simulink model "Simulinkmodel"  (R2020a)
settings: Solver=VariableStepAuto  StartTime=0.0  StopTime=10.0  RelTol=1e-3
model workspace: external: MAT-File D:\FinalSimulink\fulleasy_DataFile1.mat (data not in the file)
undefined symbols (not defined in the file or in its folder): curveData, height_plane, plane_x, plane_y, smiData, X, Y, Z
libraries: sm_lib x51, Contact_Forces_Lib x48, nesl_utility x36, walkingRobotUtils x8, simulink x1
(part 2 of 2)

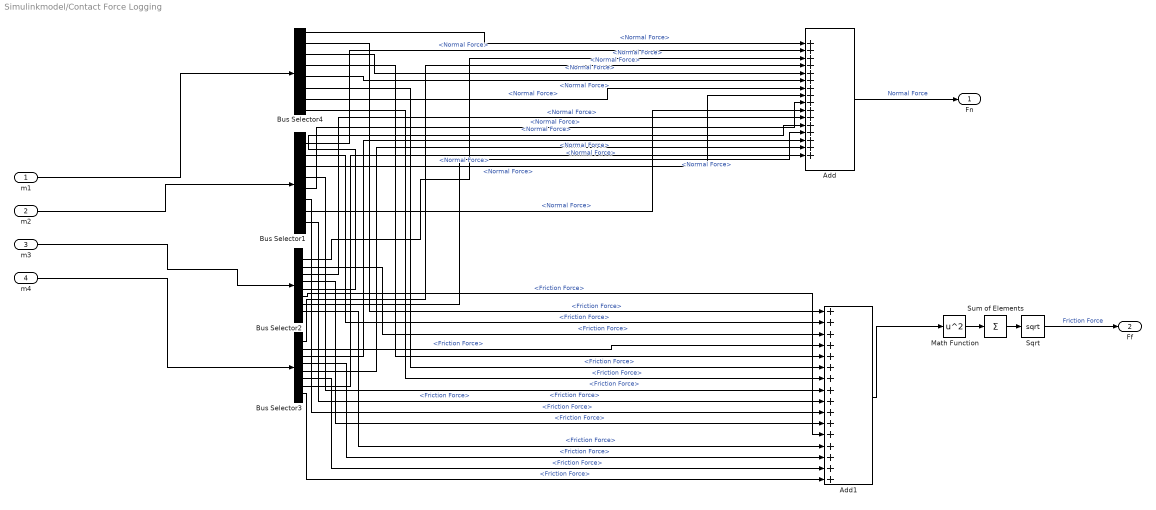
== system Simulinkmodel/Contact Force Logging ==
  m1 : Inport
  m2 : Inport  Port=2
  m3 : Inport  Port=3
  m4 : Inport  Port=4
  Add : Sum  Inputs=16
  Add1 : Sum  Inputs=16
  Bus Selector{1..4} (4 alike) : BusSelector  OutputSignals=fz1.Normal Force,fz1.Friction Force,fz2.Normal Force,fz2.Friction Force,fz3.Normal Force,fz3.Friction Force,fz4.Normal Force,fz4.Friction Force
  Math Function : Math  Operator=square  SignedPower=on  SaturateOnIntegerOverflow=on
  Sqrt : Sqrt  SaturateOnIntegerOverflow=on
  Sum of Elements : Sum  Inputs=+
  Fn : Outport  VectorParamsAs1DForOutWhenUnconnected=off
  Ff : Outport  Port=2  VectorParamsAs1DForOutWhenUnconnected=off
  wires:
  Sqrt/1 -> Ff/1  "Friction Force"
  Sum of Elements/1 -> Sqrt/1
  Math Function/1 -> Sum of Elements/1
  Add1/1 -> Math Function/1
  Add/1 -> Fn/1  "Normal Force"
  Bus Selector3/2 -> Add1/4  "<Friction Force>"
  Bus Selector2/2 -> Add1/3  "<Friction Force>"
  Bus Selector1/2 -> Add1/2  "<Friction Force>"
  Bus Selector4/2 -> Add1/1  "<Friction Force>"
  Bus Selector3/1 -> Add/4  "<Normal Force>"
  Bus Selector2/1 -> Add/3  "<Normal Force>"
  Bus Selector1/1 -> Add/2  "<Normal Force>"
  Bus Selector4/1 -> Add/1  "<Normal Force>"
  m4/1 -> Bus Selector3/1
  m3/1 -> Bus Selector2/1
  m2/1 -> Bus Selector1/1
  m1/1 -> Bus Selector4/1
  Bus Selector4/3 -> Add/5  "<Normal Force>"
  Bus Selector4/4 -> Add1/5  "<Friction Force>"
  Bus Selector4/5 -> Add/6  "<Normal Force>"
  Bus Selector4/6 -> Add1/6  "<Friction Force>"
  Bus Selector4/7 -> Add/7  "<Normal Force>"
  Bus Selector4/8 -> Add1/7  "<Friction Force>"
  Bus Selector1/3 -> Add/8  "<Normal Force>"
  Bus Selector1/4 -> Add1/8  "<Friction Force>"
  Bus Selector1/5 -> Add/9  "<Normal Force>"
  Bus Selector1/6 -> Add1/10  "<Friction Force>"
  Bus Selector1/7 -> Add/10  "<Normal Force>"
  Bus Selector1/8 -> Add1/9  "<Friction Force>"
  Bus Selector2/3 -> Add/11  "<Normal Force>"
  Bus Selector2/4 -> Add1/11  "<Friction Force>"
  Bus Selector2/5 -> Add/12  "<Normal Force>"
  Bus Selector2/6 -> Add1/12  "<Friction Force>"
  Bus Selector2/7 -> Add/13  "<Normal Force>"
  Bus Selector2/8 -> Add1/13  "<Friction Force>"
  Bus Selector3/3 -> Add/14  "<Normal Force>"
  Bus Selector3/4 -> Add1/14  "<Friction Force>"
  Bus Selector3/5 -> Add/15  "<Normal Force>"
  Bus Selector3/6 -> Add1/15  "<Friction Force>"
  Bus Selector3/7 -> Add/16  "<Normal Force>"
  Bus Selector3/8 -> Add1/16  "<Friction Force>"

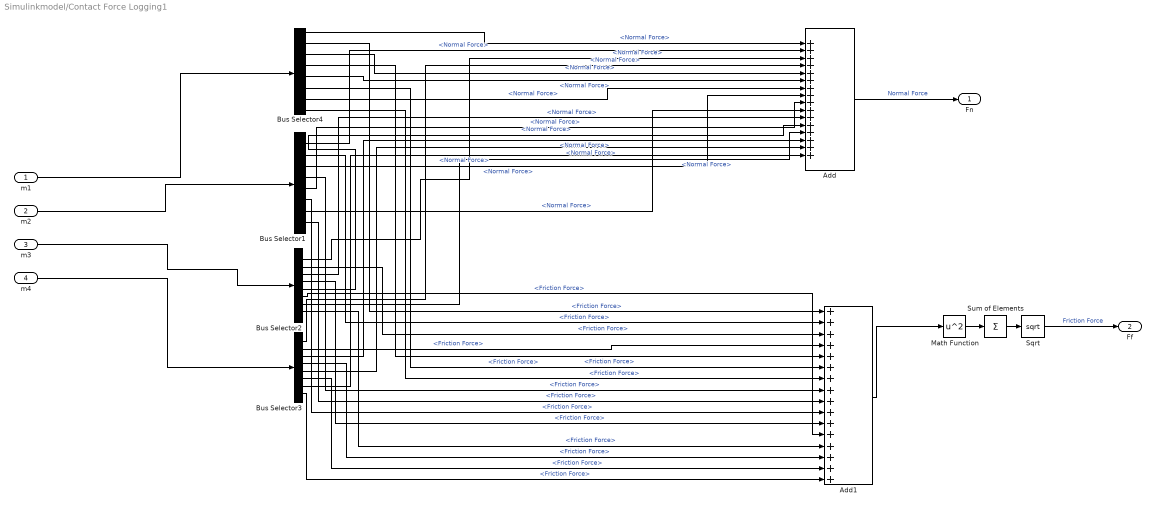
== system Simulinkmodel/Contact Force Logging1 ==
  m1 : Inport
  m2 : Inport  Port=2
  m3 : Inport  Port=3
  m4 : Inport  Port=4
  Add : Sum  Inputs=16
  Add1 : Sum  Inputs=16
  Bus Selector{1..4} (4 alike) : BusSelector  OutputSignals=fz1.Normal Force,fz1.Friction Force,fz2.Normal Force,fz2.Friction Force,fz3.Normal Force,fz3.Friction Force,fz4.Normal Force,fz4.Friction Force
  Math Function : Math  Operator=square  SignedPower=on  SaturateOnIntegerOverflow=on
  Sqrt : Sqrt  SaturateOnIntegerOverflow=on
  Sum of Elements : Sum  Inputs=+
  Fn : Outport  VectorParamsAs1DForOutWhenUnconnected=off
  Ff : Outport  Port=2  VectorParamsAs1DForOutWhenUnconnected=off
  wires:
  Bus Selector3/8 -> Add1/16  "<Friction Force>"
  Bus Selector2/5 -> Add/12  "<Normal Force>"
  Bus Selector3/6 -> Add1/15  "<Friction Force>"
  Bus Selector3/3 -> Add/14  "<Normal Force>"
  Bus Selector1/7 -> Add/10  "<Normal Force>"
  Bus Selector2/8 -> Add1/13  "<Friction Force>"
  Bus Selector3/5 -> Add/15  "<Normal Force>"
  Bus Selector1/5 -> Add/9  "<Normal Force>"
  Bus Selector2/6 -> Add1/12  "<Friction Force>"
  Bus Selector1/3 -> Add/8  "<Normal Force>"
  Bus Selector3/7 -> Add/16  "<Normal Force>"
  Bus Selector4/4 -> Add1/5  "<Friction Force>"
  Bus Selector1/4 -> Add1/8  "<Friction Force>"
  Bus Selector4/8 -> Add1/7  "<Friction Force>"
  Bus Selector1/6 -> Add1/10  "<Friction Force>"
  Bus Selector1/1 -> Add/2  "<Normal Force>"
  Bus Selector4/5 -> Add/6  "<Normal Force>"
  m2/1 -> Bus Selector1/1
  Bus Selector3/2 -> Add1/4  "<Friction Force>"
  m4/1 -> Bus Selector3/1
  Bus Selector3/1 -> Add/4  "<Normal Force>"
  Bus Selector2/1 -> Add/3  "<Normal Force>"
  Add1/1 -> Math Function/1
  Add/1 -> Fn/1  "Normal Force"
  m3/1 -> Bus Selector2/1
  Bus Selector4/1 -> Add/1  "<Normal Force>"
  Bus Selector4/2 -> Add1/1  "<Friction Force>"
  Bus Selector4/7 -> Add/7  "<Normal Force>"
  Bus Selector2/2 -> Add1/3  "<Friction Force>"
  m1/1 -> Bus Selector4/1
  Math Function/1 -> Sum of Elements/1
  Bus Selector4/6 -> Add1/6  "<Friction Force>"
  Bus Selector4/3 -> Add/5  "<Normal Force>"
  Bus Selector2/3 -> Add/11  "<Normal Force>"
  Bus Selector2/4 -> Add1/11  "<Friction Force>"
  Bus Selector1/8 -> Add1/9  "<Friction Force>"
  Sum of Elements/1 -> Sqrt/1
  Bus Selector3/4 -> Add1/14  "<Friction Force>"
  Bus Selector1/2 -> Add1/2  "<Friction Force>"
  Bus Selector2/7 -> Add/13  "<Normal Force>"
  Sqrt/1 -> Ff/1  "Friction Force"

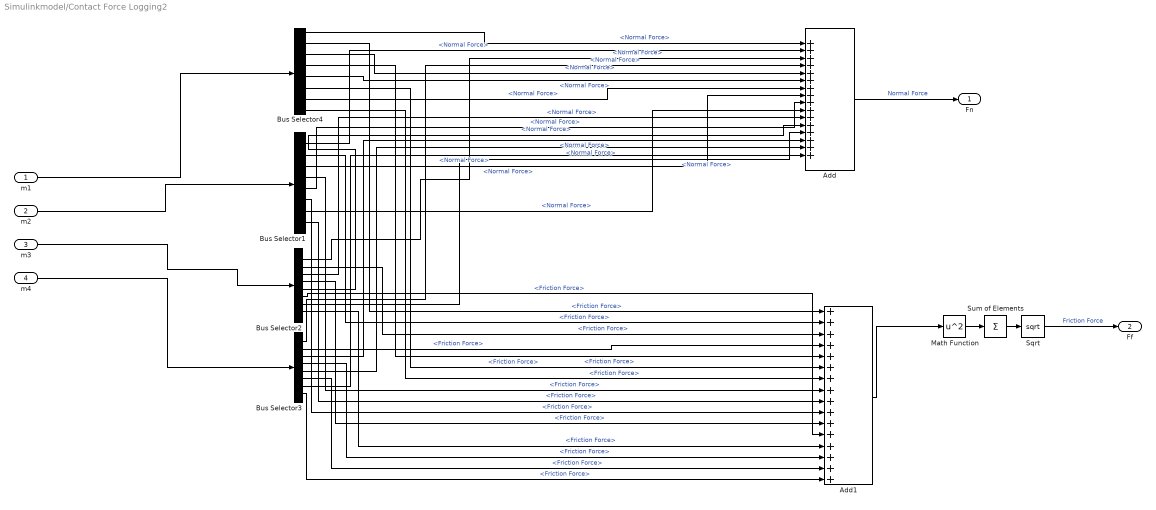
== system Simulinkmodel/Contact Force Logging2 ==
  m1 : Inport
  m2 : Inport  Port=2
  m3 : Inport  Port=3
  m4 : Inport  Port=4
  Add : Sum  Inputs=16
  Add1 : Sum  Inputs=16
  Bus Selector{1..4} (4 alike) : BusSelector  OutputSignals=fz1.Normal Force,fz1.Friction Force,fz2.Normal Force,fz2.Friction Force,fz3.Normal Force,fz3.Friction Force,fz4.Normal Force,fz4.Friction Force
  Math Function : Math  Operator=square  SignedPower=on  SaturateOnIntegerOverflow=on
  Sqrt : Sqrt  SaturateOnIntegerOverflow=on
  Sum of Elements : Sum  Inputs=+
  Fn : Outport  VectorParamsAs1DForOutWhenUnconnected=off
  Ff : Outport  Port=2  VectorParamsAs1DForOutWhenUnconnected=off
  wires:
  Bus Selector3/8 -> Add1/16  "<Friction Force>"
  Bus Selector2/5 -> Add/12  "<Normal Force>"
  Bus Selector3/6 -> Add1/15  "<Friction Force>"
  Bus Selector3/3 -> Add/14  "<Normal Force>"
  Bus Selector1/7 -> Add/10  "<Normal Force>"
  Bus Selector2/8 -> Add1/13  "<Friction Force>"
  Bus Selector3/5 -> Add/15  "<Normal Force>"
  Bus Selector1/5 -> Add/9  "<Normal Force>"
  Bus Selector2/6 -> Add1/12  "<Friction Force>"
  Bus Selector1/3 -> Add/8  "<Normal Force>"
  Bus Selector3/7 -> Add/16  "<Normal Force>"
  Bus Selector4/4 -> Add1/5  "<Friction Force>"
  Bus Selector1/4 -> Add1/8  "<Friction Force>"
  Bus Selector4/8 -> Add1/7  "<Friction Force>"
  Bus Selector1/6 -> Add1/10  "<Friction Force>"
  Bus Selector1/1 -> Add/2  "<Normal Force>"
  Bus Selector4/5 -> Add/6  "<Normal Force>"
  m2/1 -> Bus Selector1/1
  Bus Selector3/2 -> Add1/4  "<Friction Force>"
  m4/1 -> Bus Selector3/1
  Bus Selector3/1 -> Add/4  "<Normal Force>"
  Bus Selector2/1 -> Add/3  "<Normal Force>"
  Add1/1 -> Math Function/1
  Add/1 -> Fn/1  "Normal Force"
  m3/1 -> Bus Selector2/1
  Bus Selector4/1 -> Add/1  "<Normal Force>"
  Bus Selector4/2 -> Add1/1  "<Friction Force>"
  Bus Selector4/7 -> Add/7  "<Normal Force>"
  Bus Selector2/2 -> Add1/3  "<Friction Force>"
  m1/1 -> Bus Selector4/1
  Math Function/1 -> Sum of Elements/1
  Bus Selector4/6 -> Add1/6  "<Friction Force>"
  Bus Selector4/3 -> Add/5  "<Normal Force>"
  Bus Selector2/3 -> Add/11  "<Normal Force>"
  Bus Selector2/4 -> Add1/11  "<Friction Force>"
  Bus Selector1/8 -> Add1/9  "<Friction Force>"
  Sum of Elements/1 -> Sqrt/1
  Bus Selector3/4 -> Add1/14  "<Friction Force>"
  Bus Selector1/2 -> Add1/2  "<Friction Force>"
  Bus Selector2/7 -> Add/13  "<Normal Force>"
  Sqrt/1 -> Ff/1  "Friction Force"

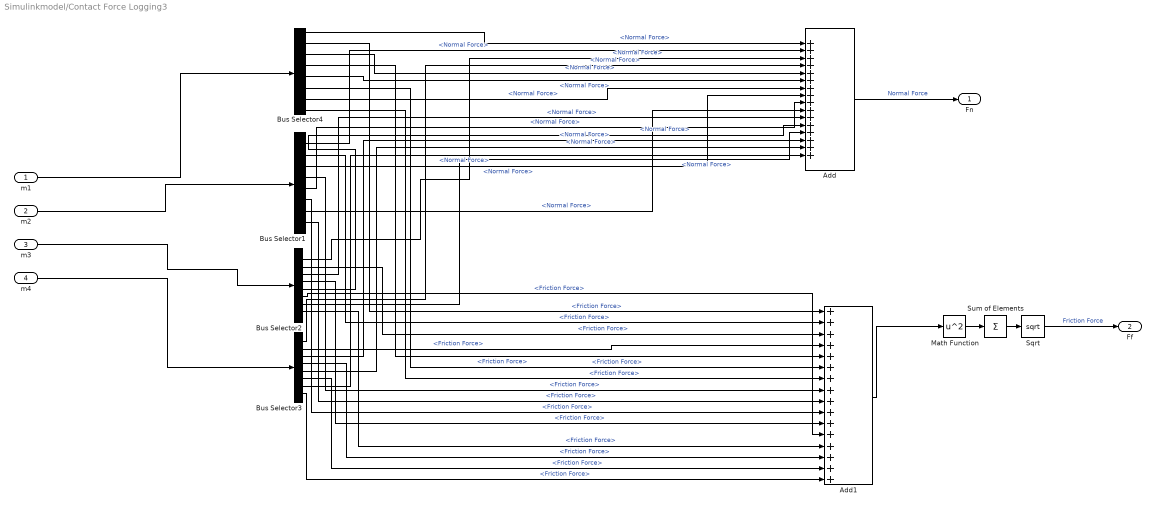
== system Simulinkmodel/Contact Force Logging3 ==
  m1 : Inport
  m2 : Inport  Port=2
  m3 : Inport  Port=3
  m4 : Inport  Port=4
  Add : Sum  Inputs=16
  Add1 : Sum  Inputs=16
  Bus Selector{1..4} (4 alike) : BusSelector  OutputSignals=fz1.Normal Force,fz1.Friction Force,fz2.Normal Force,fz2.Friction Force,fz3.Normal Force,fz3.Friction Force,fz4.Normal Force,fz4.Friction Force
  Math Function : Math  Operator=square  SignedPower=on  SaturateOnIntegerOverflow=on
  Sqrt : Sqrt  SaturateOnIntegerOverflow=on
  Sum of Elements : Sum  Inputs=+
  Fn : Outport  VectorParamsAs1DForOutWhenUnconnected=off
  Ff : Outport  Port=2  VectorParamsAs1DForOutWhenUnconnected=off
  wires:
  Bus Selector2/7 -> Add/13  "<Normal Force>"
  Bus Selector1/2 -> Add1/2  "<Friction Force>"
  Bus Selector4/6 -> Add1/6  "<Friction Force>"
  Bus Selector1/8 -> Add1/9  "<Friction Force>"
  Bus Selector2/3 -> Add/11  "<Normal Force>"
  m3/1 -> Bus Selector2/1
  m1/1 -> Bus Selector4/1
  Bus Selector4/7 -> Add/7  "<Normal Force>"
  m4/1 -> Bus Selector3/1
  Bus Selector3/1 -> Add/4  "<Normal Force>"
  Add/1 -> Fn/1  "Normal Force"
  Bus Selector3/4 -> Add1/14  "<Friction Force>"
  Add1/1 -> Math Function/1
  Bus Selector2/4 -> Add1/11  "<Friction Force>"
  Bus Selector2/1 -> Add/3  "<Normal Force>"
  Bus Selector3/2 -> Add1/4  "<Friction Force>"
  Bus Selector2/2 -> Add1/3  "<Friction Force>"
  m2/1 -> Bus Selector1/1
  Bus Selector4/1 -> Add/1  "<Normal Force>"
  Bus Selector1/6 -> Add1/10  "<Friction Force>"
  Bus Selector4/5 -> Add/6  "<Normal Force>"
  Bus Selector1/1 -> Add/2  "<Normal Force>"
  Bus Selector1/4 -> Add1/8  "<Friction Force>"
  Bus Selector4/4 -> Add1/5  "<Friction Force>"
  Sqrt/1 -> Ff/1  "Friction Force"
  Bus Selector3/7 -> Add/16  "<Normal Force>"
  Bus Selector1/3 -> Add/8  "<Normal Force>"
  Bus Selector4/3 -> Add/5  "<Normal Force>"
  Bus Selector2/8 -> Add1/13  "<Friction Force>"
  Bus Selector1/7 -> Add/10  "<Normal Force>"
  Bus Selector3/5 -> Add/15  "<Normal Force>"
  Bus Selector3/3 -> Add/14  "<Normal Force>"
  Bus Selector2/5 -> Add/12  "<Normal Force>"
  Sum of Elements/1 -> Sqrt/1
  Bus Selector3/6 -> Add1/15  "<Friction Force>"
  Bus Selector4/8 -> Add1/7  "<Friction Force>"
  Math Function/1 -> Sum of Elements/1
  Bus Selector3/8 -> Add1/16  "<Friction Force>"
  Bus Selector2/6 -> Add1/12  "<Friction Force>"
  Bus Selector4/2 -> Add1/1  "<Friction Force>"
  Bus Selector1/5 -> Add/9  "<Normal Force>"

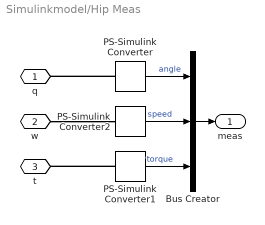
== system Simulinkmodel/Hip Meas ==
  Bus Creator : BusCreator  Inputs=3
  PS-Simulink Converter : nesl_utility/PS-Simulink Converter  PhysicalDomain=network_engine_domain  SubClassName=ps_output  LeftPortType=input  RightPortType=output  PseudoPeriodic=off  Frequencies=[]  Unit=deg  AffineConversion=off
  PS-Simulink Converter1 : nesl_utility/PS-Simulink Converter  PhysicalDomain=network_engine_domain  SubClassName=ps_output  LeftPortType=input  RightPortType=output  PseudoPeriodic=off  Frequencies=[]  Unit=N*m  AffineConversion=off
  PS-Simulink Converter2 : nesl_utility/PS-Simulink Converter  PhysicalDomain=network_engine_domain  SubClassName=ps_output  LeftPortType=input  RightPortType=output  PseudoPeriodic=off  Frequencies=[]  Unit=rad/s  AffineConversion=off
  q : PMIOPort  Side=Left
  w : PMIOPort  Port=2  Side=Left
  t : PMIOPort  Port=3  Side=Left
  meas : Outport  VectorParamsAs1DForOutWhenUnconnected=off
  wires:
  PS-Simulink Converter/1 -> Bus Creator/1  "angle"
  PS-Simulink Converter2/1 -> Bus Creator/2  "speed"
  PS-Simulink Converter1/1 -> Bus Creator/3  "torque"
  Bus Creator/1 -> meas/1
  connections:
  PS-Simulink Converter/LConn1 -- q/RConn1
  w/RConn1 -- PS-Simulink Converter2/LConn1
  PS-Simulink Converter1/LConn1 -- t/RConn1

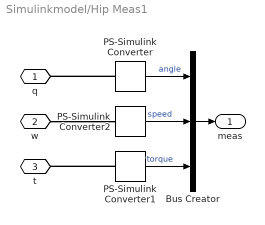
== system Simulinkmodel/Hip Meas1 ==
  Bus Creator : BusCreator  Inputs=3
  PS-Simulink Converter : nesl_utility/PS-Simulink Converter  PhysicalDomain=network_engine_domain  SubClassName=ps_output  LeftPortType=input  RightPortType=output  PseudoPeriodic=off  Frequencies=[]  Unit=deg  AffineConversion=off
  PS-Simulink Converter1 : nesl_utility/PS-Simulink Converter  PhysicalDomain=network_engine_domain  SubClassName=ps_output  LeftPortType=input  RightPortType=output  PseudoPeriodic=off  Frequencies=[]  Unit=N*m  AffineConversion=off
  PS-Simulink Converter2 : nesl_utility/PS-Simulink Converter  PhysicalDomain=network_engine_domain  SubClassName=ps_output  LeftPortType=input  RightPortType=output  PseudoPeriodic=off  Frequencies=[]  Unit=rad/s  AffineConversion=off
  q : PMIOPort  Side=Left
  w : PMIOPort  Port=2  Side=Left
  t : PMIOPort  Port=3  Side=Left
  meas : Outport  VectorParamsAs1DForOutWhenUnconnected=off
  wires:
  PS-Simulink Converter/1 -> Bus Creator/1  "angle"
  PS-Simulink Converter2/1 -> Bus Creator/2  "speed"
  PS-Simulink Converter1/1 -> Bus Creator/3  "torque"
  Bus Creator/1 -> meas/1
  connections:
  PS-Simulink Converter/LConn1 -- q/RConn1
  w/RConn1 -- PS-Simulink Converter2/LConn1
  PS-Simulink Converter1/LConn1 -- t/RConn1

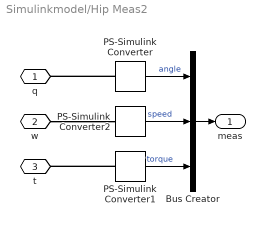
== system Simulinkmodel/Hip Meas2 ==
  Bus Creator : BusCreator  Inputs=3
  PS-Simulink Converter : nesl_utility/PS-Simulink Converter  PhysicalDomain=network_engine_domain  SubClassName=ps_output  LeftPortType=input  RightPortType=output  PseudoPeriodic=off  Frequencies=[]  Unit=deg  AffineConversion=off
  PS-Simulink Converter1 : nesl_utility/PS-Simulink Converter  PhysicalDomain=network_engine_domain  SubClassName=ps_output  LeftPortType=input  RightPortType=output  PseudoPeriodic=off  Frequencies=[]  Unit=N*m  AffineConversion=off
  PS-Simulink Converter2 : nesl_utility/PS-Simulink Converter  PhysicalDomain=network_engine_domain  SubClassName=ps_output  LeftPortType=input  RightPortType=output  PseudoPeriodic=off  Frequencies=[]  Unit=rad/s  AffineConversion=off
  q : PMIOPort  Side=Left
  w : PMIOPort  Port=2  Side=Left
  t : PMIOPort  Port=3  Side=Left
  meas : Outport  VectorParamsAs1DForOutWhenUnconnected=off
  wires:
  PS-Simulink Converter/1 -> Bus Creator/1  "angle"
  PS-Simulink Converter2/1 -> Bus Creator/2  "speed"
  PS-Simulink Converter1/1 -> Bus Creator/3  "torque"
  Bus Creator/1 -> meas/1
  connections:
  PS-Simulink Converter/LConn1 -- q/RConn1
  w/RConn1 -- PS-Simulink Converter2/LConn1
  PS-Simulink Converter1/LConn1 -- t/RConn1

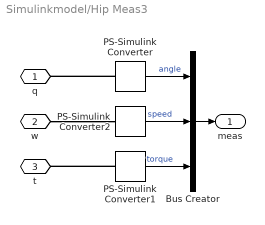
== system Simulinkmodel/Hip Meas3 ==
  Bus Creator : BusCreator  Inputs=3
  PS-Simulink Converter : nesl_utility/PS-Simulink Converter  PhysicalDomain=network_engine_domain  SubClassName=ps_output  LeftPortType=input  RightPortType=output  PseudoPeriodic=off  Frequencies=[]  Unit=deg  AffineConversion=off
  PS-Simulink Converter1 : nesl_utility/PS-Simulink Converter  PhysicalDomain=network_engine_domain  SubClassName=ps_output  LeftPortType=input  RightPortType=output  PseudoPeriodic=off  Frequencies=[]  Unit=N*m  AffineConversion=off
  PS-Simulink Converter2 : nesl_utility/PS-Simulink Converter  PhysicalDomain=network_engine_domain  SubClassName=ps_output  LeftPortType=input  RightPortType=output  PseudoPeriodic=off  Frequencies=[]  Unit=rad/s  AffineConversion=off
  q : PMIOPort  Side=Left
  w : PMIOPort  Port=2  Side=Left
  t : PMIOPort  Port=3  Side=Left
  meas : Outport  VectorParamsAs1DForOutWhenUnconnected=off
  wires:
  PS-Simulink Converter/1 -> Bus Creator/1  "angle"
  PS-Simulink Converter2/1 -> Bus Creator/2  "speed"
  PS-Simulink Converter1/1 -> Bus Creator/3  "torque"
  Bus Creator/1 -> meas/1
  connections:
  PS-Simulink Converter/LConn1 -- q/RConn1
  w/RConn1 -- PS-Simulink Converter2/LConn1
  PS-Simulink Converter1/LConn1 -- t/RConn1

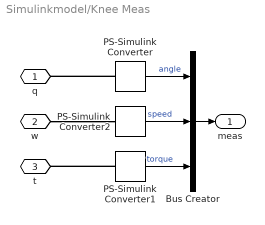
== system Simulinkmodel/Knee Meas ==
  Bus Creator : BusCreator  Inputs=3
  PS-Simulink Converter : nesl_utility/PS-Simulink Converter  PhysicalDomain=network_engine_domain  SubClassName=ps_output  LeftPortType=input  RightPortType=output  PseudoPeriodic=off  Frequencies=[]  Unit=deg  AffineConversion=off
  PS-Simulink Converter1 : nesl_utility/PS-Simulink Converter  PhysicalDomain=network_engine_domain  SubClassName=ps_output  LeftPortType=input  RightPortType=output  PseudoPeriodic=off  Frequencies=[]  Unit=N*m  AffineConversion=off
  PS-Simulink Converter2 : nesl_utility/PS-Simulink Converter  PhysicalDomain=network_engine_domain  SubClassName=ps_output  LeftPortType=input  RightPortType=output  PseudoPeriodic=off  Frequencies=[]  Unit=rad/s  AffineConversion=off
  q : PMIOPort  Side=Left
  w : PMIOPort  Port=2  Side=Left
  t : PMIOPort  Port=3  Side=Left
  meas : Outport  VectorParamsAs1DForOutWhenUnconnected=off
  wires:
  Bus Creator/1 -> meas/1
  PS-Simulink Converter1/1 -> Bus Creator/3  "torque"
  PS-Simulink Converter2/1 -> Bus Creator/2  "speed"
  PS-Simulink Converter/1 -> Bus Creator/1  "angle"
  connections:
  PS-Simulink Converter1/LConn1 -- t/RConn1
  w/RConn1 -- PS-Simulink Converter2/LConn1
  PS-Simulink Converter/LConn1 -- q/RConn1

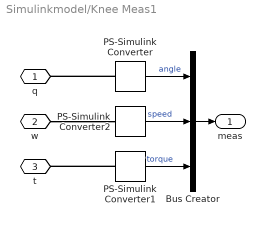
== system Simulinkmodel/Knee Meas1 ==
  Bus Creator : BusCreator  Inputs=3
  PS-Simulink Converter : nesl_utility/PS-Simulink Converter  PhysicalDomain=network_engine_domain  SubClassName=ps_output  LeftPortType=input  RightPortType=output  PseudoPeriodic=off  Frequencies=[]  Unit=deg  AffineConversion=off
  PS-Simulink Converter1 : nesl_utility/PS-Simulink Converter  PhysicalDomain=network_engine_domain  SubClassName=ps_output  LeftPortType=input  RightPortType=output  PseudoPeriodic=off  Frequencies=[]  Unit=N*m  AffineConversion=off
  PS-Simulink Converter2 : nesl_utility/PS-Simulink Converter  PhysicalDomain=network_engine_domain  SubClassName=ps_output  LeftPortType=input  RightPortType=output  PseudoPeriodic=off  Frequencies=[]  Unit=rad/s  AffineConversion=off
  q : PMIOPort  Side=Left
  w : PMIOPort  Port=2  Side=Left
  t : PMIOPort  Port=3  Side=Left
  meas : Outport  VectorParamsAs1DForOutWhenUnconnected=off
  wires:
  Bus Creator/1 -> meas/1
  PS-Simulink Converter1/1 -> Bus Creator/3  "torque"
  PS-Simulink Converter2/1 -> Bus Creator/2  "speed"
  PS-Simulink Converter/1 -> Bus Creator/1  "angle"
  connections:
  PS-Simulink Converter1/LConn1 -- t/RConn1
  w/RConn1 -- PS-Simulink Converter2/LConn1
  PS-Simulink Converter/LConn1 -- q/RConn1

== system Simulinkmodel/Knee Meas2 ==
  Bus Creator : BusCreator  Inputs=3
  PS-Simulink Converter : nesl_utility/PS-Simulink Converter  PhysicalDomain=network_engine_domain  SubClassName=ps_output  LeftPortType=input  RightPortType=output  PseudoPeriodic=off  Frequencies=[]  Unit=deg  AffineConversion=off
  PS-Simulink Converter1 : nesl_utility/PS-Simulink Converter  PhysicalDomain=network_engine_domain  SubClassName=ps_output  LeftPortType=input  RightPortType=output  PseudoPeriodic=off  Frequencies=[]  Unit=N*m  AffineConversion=off
  PS-Simulink Converter2 : nesl_utility/PS-Simulink Converter  PhysicalDomain=network_engine_domain  SubClassName=ps_output  LeftPortType=input  RightPortType=output  PseudoPeriodic=off  Frequencies=[]  Unit=rad/s  AffineConversion=off
  q : PMIOPort  Side=Left
  w : PMIOPort  Port=2  Side=Left
  t : PMIOPort  Port=3  Side=Left
  meas : Outport  VectorParamsAs1DForOutWhenUnconnected=off
  wires:
  Bus Creator/1 -> meas/1
  PS-Simulink Converter1/1 -> Bus Creator/3  "torque"
  PS-Simulink Converter2/1 -> Bus Creator/2  "speed"
  PS-Simulink Converter/1 -> Bus Creator/1  "angle"
  connections:
  PS-Simulink Converter1/LConn1 -- t/RConn1
  w/RConn1 -- PS-Simulink Converter2/LConn1
  PS-Simulink Converter/LConn1 -- q/RConn1

== system Simulinkmodel/Knee Meas3 ==
  Bus Creator : BusCreator  Inputs=3
  PS-Simulink Converter : nesl_utility/PS-Simulink Converter  PhysicalDomain=network_engine_domain  SubClassName=ps_output  LeftPortType=input  RightPortType=output  PseudoPeriodic=off  Frequencies=[]  Unit=deg  AffineConversion=off
  PS-Simulink Converter1 : nesl_utility/PS-Simulink Converter  PhysicalDomain=network_engine_domain  SubClassName=ps_output  LeftPortType=input  RightPortType=output  PseudoPeriodic=off  Frequencies=[]  Unit=N*m  AffineConversion=off
  PS-Simulink Converter2 : nesl_utility/PS-Simulink Converter  PhysicalDomain=network_engine_domain  SubClassName=ps_output  LeftPortType=input  RightPortType=output  PseudoPeriodic=off  Frequencies=[]  Unit=rad/s  AffineConversion=off
  q : PMIOPort  Side=Left
  w : PMIOPort  Port=2  Side=Left
  t : PMIOPort  Port=3  Side=Left
  meas : Outport  VectorParamsAs1DForOutWhenUnconnected=off
  wires:
  Bus Creator/1 -> meas/1
  PS-Simulink Converter1/1 -> Bus Creator/3  "torque"
  PS-Simulink Converter2/1 -> Bus Creator/2  "speed"
  PS-Simulink Converter/1 -> Bus Creator/1  "angle"
  connections:
  PS-Simulink Converter1/LConn1 -- t/RConn1
  w/RConn1 -- PS-Simulink Converter2/LConn1
  PS-Simulink Converter/LConn1 -- q/RConn1

== system Simulinkmodel/Package Measurements ==
  Fn : Inport
  Ff : Inport  Port=2
  knee : Inport  Port=3
  hip : Inport  Port=4
  Bus Creator3 : BusCreator  Inputs=8
  Extract Measurements1 : Subsystem
  Extract Measurements2 : Subsystem
  meas : Outport  VectorParamsAs1DForOutWhenUnconnected=off
  wires:
  Fn/1 -> Bus Creator3/1  "normal_force"
  Ff/1 -> Bus Creator3/2  "friction_force"
  Extract Measurements2/2(torque) -> Bus Creator3/8  "hip_torque"
  Extract Measurements2/1(angle) -> Bus Creator3/7  "hip_angle"
  Extract Measurements1/2(torque) -> Bus Creator3/6  "knee_torque"
  Extract Measurements1/1(angle) -> Bus Creator3/5  "knee_angle"
  hip/1 -> Extract Measurements2/1(meas)
  knee/1 -> Extract Measurements1/1(meas)
  Bus Creator3/1 -> meas/1

== system Simulinkmodel/Package Measurements1 ==
  Fn : Inport
  Ff : Inport  Port=2
  knee : Inport  Port=3
  hip : Inport  Port=4
  Bus Creator3 : BusCreator  Inputs=8
  Extract Measurements1 : Subsystem
  Extract Measurements2 : Subsystem
  meas : Outport  VectorParamsAs1DForOutWhenUnconnected=off
  wires:
  Fn/1 -> Bus Creator3/1  "normal_force"
  Ff/1 -> Bus Creator3/2  "friction_force"
  Extract Measurements2/2(torque) -> Bus Creator3/8  "hip_torque"
  Extract Measurements2/1(angle) -> Bus Creator3/7  "hip_angle"
  Extract Measurements1/2(torque) -> Bus Creator3/6  "knee_torque"
  Extract Measurements1/1(angle) -> Bus Creator3/5  "knee_angle"
  hip/1 -> Extract Measurements2/1(meas)
  knee/1 -> Extract Measurements1/1(meas)
  Bus Creator3/1 -> meas/1

== system Simulinkmodel/Package Measurements2 ==
  Fn : Inport
  Ff : Inport  Port=2
  knee : Inport  Port=3
  hip : Inport  Port=4
  Bus Creator3 : BusCreator  Inputs=8
  Extract Measurements1 : Subsystem
  Extract Measurements2 : Subsystem
  meas : Outport  VectorParamsAs1DForOutWhenUnconnected=off
  wires:
  Fn/1 -> Bus Creator3/1  "normal_force"
  Ff/1 -> Bus Creator3/2  "friction_force"
  Extract Measurements2/2(torque) -> Bus Creator3/8  "hip_torque"
  Extract Measurements2/1(angle) -> Bus Creator3/7  "hip_angle"
  Extract Measurements1/2(torque) -> Bus Creator3/6  "knee_torque"
  Extract Measurements1/1(angle) -> Bus Creator3/5  "knee_angle"
  hip/1 -> Extract Measurements2/1(meas)
  knee/1 -> Extract Measurements1/1(meas)
  Bus Creator3/1 -> meas/1

== system Simulinkmodel/Package Measurements3 ==
  Fn : Inport
  Ff : Inport  Port=2
  knee : Inport  Port=3
  hip : Inport  Port=4
  Bus Creator3 : BusCreator  Inputs=8
  Extract Measurements1 : Subsystem
  Extract Measurements2 : Subsystem
  meas : Outport  VectorParamsAs1DForOutWhenUnconnected=off
  wires:
  Fn/1 -> Bus Creator3/1  "normal_force"
  Ff/1 -> Bus Creator3/2  "friction_force"
  Extract Measurements2/2(torque) -> Bus Creator3/8  "hip_torque"
  Extract Measurements2/1(angle) -> Bus Creator3/7  "hip_angle"
  Extract Measurements1/2(torque) -> Bus Creator3/6  "knee_torque"
  Extract Measurements1/1(angle) -> Bus Creator3/5  "knee_angle"
  hip/1 -> Extract Measurements2/1(meas)
  knee/1 -> Extract Measurements1/1(meas)
  Bus Creator3/1 -> meas/1

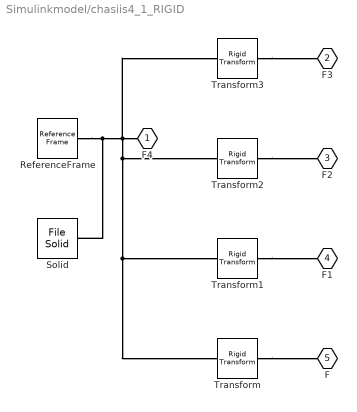
== system Simulinkmodel/chasiis4_1_RIGID ==
  ReferenceFrame : sm_lib/Frames and Transforms/Reference Frame
  Solid : sm_lib/Body Elements/File Solid  ExtGeomFileName=D:\FinalSimulink\STEPFILES\chassisbasic.STEP  UnitType=FromFile  ExtGeomFileUnits=m  StepReaderType=HEX  ExportConvexHullGeometry=off  InertiaType=Custom  Mass=smiData.Solid(2).mass  MassUnits=kg  CenterOfMass=smiData.Solid(2).CoM  CenterOfMassUnits=mm  MomentsOfInertia=smiData.Solid(2).MoI  MomentsOfInertiaUnits=kg*mm^2  ProductsOfInertia=smiData.Solid(2).PoI  ProductsOfInertiaUnits=kg*mm^2  BasedOnType=Density  Density=1000  DensityUnits=kg/m^3  DoExposeReferenceFrame=on  SerializedFrames=<Frames/>  GraphicType=FromGeometry  MarkerShape=Sphere  MarkerSize=10  GraphicVisPropType=SimpleVisualProperties  GraphicDiffuseColor=smiData.Solid(2).color  GraphicSpecularColor=[0.5 0.5 0.5 1.0]  GraphicAmbientColor=[0.15 0.15 0.15 1.0]  GraphicEmissiveColor=[0.0 0.0 0.0 1.0]  GraphicShininess=75  GraphicOpacity=smiData.Solid(2).opacity
  Transform : sm_lib/Frames and Transforms/Rigid Transform  TranslationMethod=Cartesian  TranslationStandardOffset=0  TranslationLengthUnit=mm  TranslationStandardAxis=+Z  TranslationCartesianOffset=smiData.RigidTransform(1).translation  TranslationROffset=0  TranslationROffsetUnits=m  TranslationZOffset=0  TranslationZOffsetUnits=m  TranslationThetaOffset=0  TranslationThetaOffsetUnits=deg  RotationMethod=ArbitraryAxis  RotationAngleUnits=rad  RotationStandardAxis=+Z  RotationAngle=smiData.RigidTransform(1).angle  RotationArbitraryAxis=smiData.RigidTransform(1).axis  FollAlignAxisA=+X  BaseAlignAxisA=+Y  FollAlignAxisB=+Y  BaseAlignAxisB=+Z  RotationSequenceAxes=FollowerAxes  RotationSequence=XYX  RotationSequenceAngles=[0 0 0]  RotationSequenceAnglesUnits=deg  RotationMatrix=[1 0 0; 0 1 0; 0 0 1]
  Transform1 : sm_lib/Frames and Transforms/Rigid Transform  TranslationMethod=Cartesian  TranslationStandardOffset=0  TranslationLengthUnit=mm  TranslationStandardAxis=+Z  TranslationCartesianOffset=smiData.RigidTransform(5).translation  TranslationROffset=0  TranslationROffsetUnits=m  TranslationZOffset=0  TranslationZOffsetUnits=m  TranslationThetaOffset=0  TranslationThetaOffsetUnits=deg  RotationMethod=ArbitraryAxis  RotationAngleUnits=rad  RotationStandardAxis=+Z  RotationAngle=smiData.RigidTransform(5).angle  RotationArbitraryAxis=smiData.RigidTransform(5).axis  FollAlignAxisA=+X  BaseAlignAxisA=+Y  FollAlignAxisB=+Y  BaseAlignAxisB=+Z  RotationSequenceAxes=FollowerAxes  RotationSequence=XYX  RotationSequenceAngles=[0 0 0]  RotationSequenceAnglesUnits=deg  RotationMatrix=[1 0 0; 0 1 0; 0 0 1]
  Transform2 : sm_lib/Frames and Transforms/Rigid Transform  TranslationMethod=Cartesian  TranslationStandardOffset=0  TranslationLengthUnit=mm  TranslationStandardAxis=+Z  TranslationCartesianOffset=smiData.RigidTransform(9).translation  TranslationROffset=0  TranslationROffsetUnits=m  TranslationZOffset=0  TranslationZOffsetUnits=m  TranslationThetaOffset=0  TranslationThetaOffsetUnits=deg  RotationMethod=ArbitraryAxis  RotationAngleUnits=rad  RotationStandardAxis=+Z  RotationAngle=smiData.RigidTransform(9).angle  RotationArbitraryAxis=smiData.RigidTransform(9).axis  FollAlignAxisA=+X  BaseAlignAxisA=+Y  FollAlignAxisB=+Y  BaseAlignAxisB=+Z  RotationSequenceAxes=FollowerAxes  RotationSequence=XYX  RotationSequenceAngles=[0 0 0]  RotationSequenceAnglesUnits=deg  RotationMatrix=[1 0 0; 0 1 0; 0 0 1]
  Transform3 : sm_lib/Frames and Transforms/Rigid Transform  TranslationMethod=Cartesian  TranslationStandardOffset=0  TranslationLengthUnit=mm  TranslationStandardAxis=+Z  TranslationCartesianOffset=smiData.RigidTransform(13).translation  TranslationROffset=0  TranslationROffsetUnits=m  TranslationZOffset=0  TranslationZOffsetUnits=m  TranslationThetaOffset=0  TranslationThetaOffsetUnits=deg  RotationMethod=ArbitraryAxis  RotationAngleUnits=rad  RotationStandardAxis=+Z  RotationAngle=smiData.RigidTransform(13).angle  RotationArbitraryAxis=smiData.RigidTransform(13).axis  FollAlignAxisA=+X  BaseAlignAxisA=+Y  FollAlignAxisB=+Y  BaseAlignAxisB=+Z  RotationSequenceAxes=FollowerAxes  RotationSequence=XYX  RotationSequenceAngles=[0 0 0]  RotationSequenceAnglesUnits=deg  RotationMatrix=[1 0 0; 0 1 0; 0 0 1]
  F4 : PMIOPort  Side=Left
  F3 : PMIOPort  Port=2  Side=Right
  F2 : PMIOPort  Port=3  Side=Right
  F1 : PMIOPort  Port=4  Side=Right
  F : PMIOPort  Port=5  Side=Right
  connections:
  Solid/RConn1 -- ReferenceFrame/RConn1 -- Transform/LConn1 -- Transform1/LConn1 -- Transform2/LConn1 -- Transform3/LConn1 -- F4/RConn1
  Transform/RConn1 -- F/RConn1
  Transform1/RConn1 -- F1/RConn1
  Transform2/RConn1 -- F2/RConn1
  Transform3/RConn1 -- F3/RConn1

== system Simulinkmodel/thigh2_7_RIGID ==
  ReferenceFrame : sm_lib/Frames and Transforms/Reference Frame
  Solid : sm_lib/Body Elements/File Solid  ExtGeomFileName=D:\FinalSimulink\STEPFILES\thigh2_Default_sldprt.STEP  UnitType=FromFile  ExtGeomFileUnits=m  StepReaderType=HEX  ExportConvexHullGeometry=off  InertiaType=Custom  Mass=smiData.Solid(3).mass  MassUnits=kg  CenterOfMass=smiData.Solid(3).CoM  CenterOfMassUnits=mm  MomentsOfInertia=smiData.Solid(3).MoI  MomentsOfInertiaUnits=kg*mm^2  ProductsOfInertia=smiData.Solid(3).PoI  ProductsOfInertiaUnits=kg*mm^2  BasedOnType=Density  Density=1000  DensityUnits=kg/m^3  DoExposeReferenceFrame=on  SerializedFrames=<Frames/>  GraphicType=FromGeometry  MarkerShape=Sphere  MarkerSize=10  GraphicVisPropType=SimpleVisualProperties  GraphicDiffuseColor=smiData.Solid(3).color  GraphicSpecularColor=[0.5 0.5 0.5 1.0]  GraphicAmbientColor=[0.15 0.15 0.15 1.0]  GraphicEmissiveColor=[0.0 0.0 0.0 1.0]  GraphicShininess=75  GraphicOpacity=smiData.Solid(3).opacity
  Transform : sm_lib/Frames and Transforms/Rigid Transform  TranslationMethod=Cartesian  TranslationStandardOffset=0  TranslationLengthUnit=mm  TranslationStandardAxis=+Z  TranslationCartesianOffset=smiData.RigidTransform(14).translation  TranslationROffset=0  TranslationROffsetUnits=m  TranslationZOffset=0  TranslationZOffsetUnits=m  TranslationThetaOffset=0  TranslationThetaOffsetUnits=deg  RotationMethod=ArbitraryAxis  RotationAngleUnits=rad  RotationStandardAxis=+Z  RotationAngle=smiData.RigidTransform(2).angle  RotationArbitraryAxis=smiData.RigidTransform(2).axis  FollAlignAxisA=+X  BaseAlignAxisA=+Y  FollAlignAxisB=+Y  BaseAlignAxisB=+Z  RotationSequenceAxes=FollowerAxes  RotationSequence=XYX  RotationSequenceAngles=[0 0 0]  RotationSequenceAnglesUnits=deg  RotationMatrix=[1 0 0; 0 1 0; 0 0 1]
  Transform1 : sm_lib/Frames and Transforms/Rigid Transform  TranslationMethod=Cartesian  TranslationStandardOffset=0  TranslationLengthUnit=mm  TranslationStandardAxis=+Z  TranslationCartesianOffset=smiData.RigidTransform(16).translation  TranslationROffset=0  TranslationROffsetUnits=m  TranslationZOffset=0  TranslationZOffsetUnits=m  TranslationThetaOffset=0  TranslationThetaOffsetUnits=deg  RotationMethod=ArbitraryAxis  RotationAngleUnits=rad  RotationStandardAxis=+Z  RotationAngle=smiData.RigidTransform(3).angle  RotationArbitraryAxis=smiData.RigidTransform(3).axis  FollAlignAxisA=+X  BaseAlignAxisA=+Y  FollAlignAxisB=+Y  BaseAlignAxisB=+Z  RotationSequenceAxes=FollowerAxes  RotationSequence=XYX  RotationSequenceAngles=[0 0 0]  RotationSequenceAnglesUnits=deg  RotationMatrix=[1 0 0; 0 1 0; 0 0 1]
  F1 : PMIOPort  Side=Left
  F : PMIOPort  Port=2  Side=Left
  connections:
  Solid/RConn1 -- ReferenceFrame/RConn1 -- Transform/LConn1 -- Transform1/LConn1
  Transform/RConn1 -- F/RConn1
  Transform1/RConn1 -- F1/RConn1

== system Simulinkmodel/thigh2_7_RIGID1 ==
  ReferenceFrame : sm_lib/Frames and Transforms/Reference Frame
  Solid : sm_lib/Body Elements/File Solid  ExtGeomFileName=D:\FinalSimulink\STEPFILES\thigh2_Default_sldprt.STEP  UnitType=FromFile  ExtGeomFileUnits=m  StepReaderType=HEX  ExportConvexHullGeometry=off  InertiaType=Custom  Mass=smiData.Solid(3).mass  MassUnits=kg  CenterOfMass=smiData.Solid(3).CoM  CenterOfMassUnits=mm  MomentsOfInertia=smiData.Solid(3).MoI  MomentsOfInertiaUnits=kg*mm^2  ProductsOfInertia=smiData.Solid(3).PoI  ProductsOfInertiaUnits=kg*mm^2  BasedOnType=Density  Density=1000  DensityUnits=kg/m^3  DoExposeReferenceFrame=on  SerializedFrames=<Frames/>  GraphicType=FromGeometry  MarkerShape=Sphere  MarkerSize=10  GraphicVisPropType=SimpleVisualProperties  GraphicDiffuseColor=smiData.Solid(3).color  GraphicSpecularColor=[0.5 0.5 0.5 1.0]  GraphicAmbientColor=[0.15 0.15 0.15 1.0]  GraphicEmissiveColor=[0.0 0.0 0.0 1.0]  GraphicShininess=75  GraphicOpacity=smiData.Solid(3).opacity
  Transform : sm_lib/Frames and Transforms/Rigid Transform  TranslationMethod=Cartesian  TranslationStandardOffset=0  TranslationLengthUnit=mm  TranslationStandardAxis=+Z  TranslationCartesianOffset=smiData.RigidTransform(14).translation  TranslationROffset=0  TranslationROffsetUnits=m  TranslationZOffset=0  TranslationZOffsetUnits=m  TranslationThetaOffset=0  TranslationThetaOffsetUnits=deg  RotationMethod=ArbitraryAxis  RotationAngleUnits=rad  RotationStandardAxis=+Z  RotationAngle=smiData.RigidTransform(6).angle  RotationArbitraryAxis=smiData.RigidTransform(6).axis  FollAlignAxisA=+X  BaseAlignAxisA=+Y  FollAlignAxisB=+Y  BaseAlignAxisB=+Z  RotationSequenceAxes=FollowerAxes  RotationSequence=XYX  RotationSequenceAngles=[0 0 0]  RotationSequenceAnglesUnits=deg  RotationMatrix=[1 0 0; 0 1 0; 0 0 1]
  Transform1 : sm_lib/Frames and Transforms/Rigid Transform  TranslationMethod=Cartesian  TranslationStandardOffset=0  TranslationLengthUnit=mm  TranslationStandardAxis=+Z  TranslationCartesianOffset=smiData.RigidTransform(16).translation  TranslationROffset=0  TranslationROffsetUnits=m  TranslationZOffset=0  TranslationZOffsetUnits=m  TranslationThetaOffset=0  TranslationThetaOffsetUnits=deg  RotationMethod=ArbitraryAxis  RotationAngleUnits=rad  RotationStandardAxis=+Z  RotationAngle=smiData.RigidTransform(7).angle  RotationArbitraryAxis=smiData.RigidTransform(7).axis  FollAlignAxisA=+X  BaseAlignAxisA=+Y  FollAlignAxisB=+Y  BaseAlignAxisB=+Z  RotationSequenceAxes=FollowerAxes  RotationSequence=XYX  RotationSequenceAngles=[0 0 0]  RotationSequenceAnglesUnits=deg  RotationMatrix=[1 0 0; 0 1 0; 0 0 1]
  F1 : PMIOPort  Side=Left
  F : PMIOPort  Port=2  Side=Left
  connections:
  Transform/LConn1 -- Transform1/LConn1 -- ReferenceFrame/RConn1 -- Solid/RConn1
  Transform/RConn1 -- F/RConn1
  Transform1/RConn1 -- F1/RConn1

== system Simulinkmodel/thigh2_7_RIGID2 ==
  ReferenceFrame : sm_lib/Frames and Transforms/Reference Frame
  Solid : sm_lib/Body Elements/File Solid  ExtGeomFileName=D:\FinalSimulink\STEPFILES\thigh2_Default_sldprt.STEP  UnitType=FromFile  ExtGeomFileUnits=m  StepReaderType=HEX  ExportConvexHullGeometry=off  InertiaType=Custom  Mass=smiData.Solid(3).mass  MassUnits=kg  CenterOfMass=smiData.Solid(3).CoM  CenterOfMassUnits=mm  MomentsOfInertia=smiData.Solid(3).MoI  MomentsOfInertiaUnits=kg*mm^2  ProductsOfInertia=smiData.Solid(3).PoI  ProductsOfInertiaUnits=kg*mm^2  BasedOnType=Density  Density=1000  DensityUnits=kg/m^3  DoExposeReferenceFrame=on  SerializedFrames=<Frames/>  GraphicType=FromGeometry  MarkerShape=Sphere  MarkerSize=10  GraphicVisPropType=SimpleVisualProperties  GraphicDiffuseColor=smiData.Solid(3).color  GraphicSpecularColor=[0.5 0.5 0.5 1.0]  GraphicAmbientColor=[0.15 0.15 0.15 1.0]  GraphicEmissiveColor=[0.0 0.0 0.0 1.0]  GraphicShininess=75  GraphicOpacity=smiData.Solid(3).opacity
  Transform : sm_lib/Frames and Transforms/Rigid Transform  TranslationMethod=Cartesian  TranslationStandardOffset=0  TranslationLengthUnit=mm  TranslationStandardAxis=+Z  TranslationCartesianOffset=smiData.RigidTransform(14).translation  TranslationROffset=0  TranslationROffsetUnits=m  TranslationZOffset=0  TranslationZOffsetUnits=m  TranslationThetaOffset=0  TranslationThetaOffsetUnits=deg  RotationMethod=ArbitraryAxis  RotationAngleUnits=rad  RotationStandardAxis=+Z  RotationAngle=smiData.RigidTransform(10).angle  RotationArbitraryAxis=smiData.RigidTransform(10).axis  FollAlignAxisA=+X  BaseAlignAxisA=+Y  FollAlignAxisB=+Y  BaseAlignAxisB=+Z  RotationSequenceAxes=FollowerAxes  RotationSequence=XYX  RotationSequenceAngles=[0 0 0]  RotationSequenceAnglesUnits=deg  RotationMatrix=[1 0 0; 0 1 0; 0 0 1]
  Transform1 : sm_lib/Frames and Transforms/Rigid Transform  TranslationMethod=Cartesian  TranslationStandardOffset=0  TranslationLengthUnit=mm  TranslationStandardAxis=+Z  TranslationCartesianOffset=smiData.RigidTransform(16).translation  TranslationROffset=0  TranslationROffsetUnits=m  TranslationZOffset=0  TranslationZOffsetUnits=m  TranslationThetaOffset=0  TranslationThetaOffsetUnits=deg  RotationMethod=ArbitraryAxis  RotationAngleUnits=rad  RotationStandardAxis=+Z  RotationAngle=smiData.RigidTransform(11).angle  RotationArbitraryAxis=smiData.RigidTransform(11).axis  FollAlignAxisA=+X  BaseAlignAxisA=+Y  FollAlignAxisB=+Y  BaseAlignAxisB=+Z  RotationSequenceAxes=FollowerAxes  RotationSequence=XYX  RotationSequenceAngles=[0 0 0]  RotationSequenceAnglesUnits=deg  RotationMatrix=[1 0 0; 0 1 0; 0 0 1]
  F1 : PMIOPort  Side=Left
  F : PMIOPort  Port=2  Side=Left
  connections:
  Transform/LConn1 -- Transform1/LConn1 -- ReferenceFrame/RConn1 -- Solid/RConn1
  Transform/RConn1 -- F/RConn1
  Transform1/RConn1 -- F1/RConn1

== system Simulinkmodel/thigh2_7_RIGID3 ==
  ReferenceFrame : sm_lib/Frames and Transforms/Reference Frame
  Solid : sm_lib/Body Elements/File Solid  ExtGeomFileName=D:\FinalSimulink\STEPFILES\thigh2_Default_sldprt.STEP  UnitType=FromFile  ExtGeomFileUnits=m  StepReaderType=HEX  ExportConvexHullGeometry=off  InertiaType=Custom  Mass=smiData.Solid(3).mass  MassUnits=kg  CenterOfMass=smiData.Solid(3).CoM  CenterOfMassUnits=mm  MomentsOfInertia=smiData.Solid(3).MoI  MomentsOfInertiaUnits=kg*mm^2  ProductsOfInertia=smiData.Solid(3).PoI  ProductsOfInertiaUnits=kg*mm^2  BasedOnType=Density  Density=1000  DensityUnits=kg/m^3  DoExposeReferenceFrame=on  SerializedFrames=<Frames/>  GraphicType=FromGeometry  MarkerShape=Sphere  MarkerSize=10  GraphicVisPropType=SimpleVisualProperties  GraphicDiffuseColor=smiData.Solid(3).color  GraphicSpecularColor=[0.5 0.5 0.5 1.0]  GraphicAmbientColor=[0.15 0.15 0.15 1.0]  GraphicEmissiveColor=[0.0 0.0 0.0 1.0]  GraphicShininess=75  GraphicOpacity=smiData.Solid(3).opacity
  Transform : sm_lib/Frames and Transforms/Rigid Transform  TranslationMethod=Cartesian  TranslationStandardOffset=0  TranslationLengthUnit=mm  TranslationStandardAxis=+Z  TranslationCartesianOffset=smiData.RigidTransform(14).translation  TranslationROffset=0  TranslationROffsetUnits=m  TranslationZOffset=0  TranslationZOffsetUnits=m  TranslationThetaOffset=0  TranslationThetaOffsetUnits=deg  RotationMethod=ArbitraryAxis  RotationAngleUnits=rad  RotationStandardAxis=+Z  RotationAngle=smiData.RigidTransform(14).angle  RotationArbitraryAxis=smiData.RigidTransform(14).axis  FollAlignAxisA=+X  BaseAlignAxisA=+Y  FollAlignAxisB=+Y  BaseAlignAxisB=+Z  RotationSequenceAxes=FollowerAxes  RotationSequence=XYX  RotationSequenceAngles=[0 0 0]  RotationSequenceAnglesUnits=deg  RotationMatrix=[1 0 0; 0 1 0; 0 0 1]
  Transform1 : sm_lib/Frames and Transforms/Rigid Transform  TranslationMethod=Cartesian  TranslationStandardOffset=0  TranslationLengthUnit=mm  TranslationStandardAxis=+Z  TranslationCartesianOffset=smiData.RigidTransform(16).translation  TranslationROffset=0  TranslationROffsetUnits=m  TranslationZOffset=0  TranslationZOffsetUnits=m  TranslationThetaOffset=0  TranslationThetaOffsetUnits=deg  RotationMethod=ArbitraryAxis  RotationAngleUnits=rad  RotationStandardAxis=+Z  RotationAngle=smiData.RigidTransform(16).angle  RotationArbitraryAxis=smiData.RigidTransform(16).axis  FollAlignAxisA=+X  BaseAlignAxisA=+Y  FollAlignAxisB=+Y  BaseAlignAxisB=+Z  RotationSequenceAxes=FollowerAxes  RotationSequence=XYX  RotationSequenceAngles=[0 0 0]  RotationSequenceAnglesUnits=deg  RotationMatrix=[1 0 0; 0 1 0; 0 0 1]
  F1 : PMIOPort  Side=Left
  F : PMIOPort  Port=2  Side=Left
  connections:
  Transform/LConn1 -- Transform1/LConn1 -- ReferenceFrame/RConn1 -- Solid/RConn1
  Transform/RConn1 -- F/RConn1
  Transform1/RConn1 -- F1/RConn1

== system Simulinkmodel/Package Measurements/Extract Measurements1 ==
  meas : Inport
  Bus Selector : BusSelector  OutputSignals=angle,torque
  angle : Outport  VectorParamsAs1DForOutWhenUnconnected=off
  torque : Outport  Port=2  VectorParamsAs1DForOutWhenUnconnected=off
  wires:
  Bus Selector/2 -> torque/1  "<torque>"
  meas/1 -> Bus Selector/1
  Bus Selector/1 -> angle/1  "<angle>"

== system Simulinkmodel/Package Measurements/Extract Measurements2 ==
  meas : Inport
  Bus Selector : BusSelector  OutputSignals=angle,torque
  angle : Outport  VectorParamsAs1DForOutWhenUnconnected=off
  torque : Outport  Port=2  VectorParamsAs1DForOutWhenUnconnected=off
  wires:
  Bus Selector/1 -> angle/1  "<angle>"
  meas/1 -> Bus Selector/1
  Bus Selector/2 -> torque/1  "<torque>"

== system Simulinkmodel/Package Measurements1/Extract Measurements1 ==
  meas : Inport
  Bus Selector : BusSelector  OutputSignals=angle,torque
  angle : Outport  VectorParamsAs1DForOutWhenUnconnected=off
  torque : Outport  Port=2  VectorParamsAs1DForOutWhenUnconnected=off
  wires:
  Bus Selector/2 -> torque/1  "<torque>"
  meas/1 -> Bus Selector/1
  Bus Selector/1 -> angle/1  "<angle>"

== system Simulinkmodel/Package Measurements1/Extract Measurements2 ==
  meas : Inport
  Bus Selector : BusSelector  OutputSignals=angle,torque
  angle : Outport  VectorParamsAs1DForOutWhenUnconnected=off
  torque : Outport  Port=2  VectorParamsAs1DForOutWhenUnconnected=off
  wires:
  Bus Selector/1 -> angle/1  "<angle>"
  meas/1 -> Bus Selector/1
  Bus Selector/2 -> torque/1  "<torque>"

== system Simulinkmodel/Package Measurements2/Extract Measurements1 ==
  meas : Inport
  Bus Selector : BusSelector  OutputSignals=angle,torque
  angle : Outport  VectorParamsAs1DForOutWhenUnconnected=off
  torque : Outport  Port=2  VectorParamsAs1DForOutWhenUnconnected=off
  wires:
  Bus Selector/2 -> torque/1  "<torque>"
  meas/1 -> Bus Selector/1
  Bus Selector/1 -> angle/1  "<angle>"

== system Simulinkmodel/Package Measurements2/Extract Measurements2 ==
  meas : Inport
  Bus Selector : BusSelector  OutputSignals=angle,torque
  angle : Outport  VectorParamsAs1DForOutWhenUnconnected=off
  torque : Outport  Port=2  VectorParamsAs1DForOutWhenUnconnected=off
  wires:
  Bus Selector/1 -> angle/1  "<angle>"
  meas/1 -> Bus Selector/1
  Bus Selector/2 -> torque/1  "<torque>"

== system Simulinkmodel/Package Measurements3/Extract Measurements1 ==
  meas : Inport
  Bus Selector : BusSelector  OutputSignals=angle,torque
  angle : Outport  VectorParamsAs1DForOutWhenUnconnected=off
  torque : Outport  Port=2  VectorParamsAs1DForOutWhenUnconnected=off
  wires:
  Bus Selector/2 -> torque/1  "<torque>"
  meas/1 -> Bus Selector/1
  Bus Selector/1 -> angle/1  "<angle>"

== system Simulinkmodel/Package Measurements3/Extract Measurements2 ==
  meas : Inport
  Bus Selector : BusSelector  OutputSignals=angle,torque
  angle : Outport  VectorParamsAs1DForOutWhenUnconnected=off
  torque : Outport  Port=2  VectorParamsAs1DForOutWhenUnconnected=off
  wires:
  Bus Selector/1 -> angle/1  "<angle>"
  meas/1 -> Bus Selector/1
  Bus Selector/2 -> torque/1  "<torque>"
